simulink model "H2DFRL_LExCI_env_PPO"  (R2023a)
settings: Solver=FixedStepAuto  StartTime=0.0  StopTime=50  FixedStep=0.08  RelTol=1e-3
values from neighbouring files (symbols this model uses):
  action_mean_selector_ppo = 1:num_actions    [ReinforcementLearningBlockInit_H2DFRL.m]
  action_sampling_mode = 1    [ReinforcementLearningBlockInit_H2DFRL.m]
  action_selector_ddpg = 1:num_actions    [ReinforcementLearningBlockInit_H2DFRL.m]
  action_std_selector_ppo = 1:num_actions    [ReinforcementLearningBlockInit_H2DFRL.m]
  action_type = 1    [ReinforcementLearningBlockInit_H2DFRL.m]
  C2C_NMPC = init_C2C_NMPC_H2DF(C2C_NMPC.expdata)    [init_H2DFRL_GRU.m]
  LowerLimit = ([0.17e-3;350;-5;1e-3] - C2C_NMPC.Normalization.controls.mean)./(C2C_NMPC.Normalization.controls.std)    [init_H2DFRL_GRU.m]
  num_actions = 4    [ReinforcementLearningBlockInit_H2DFRL.m]
  rl_algorithm = 1    [ReinforcementLearningBlockInit_H2DFRL.m]
  UpperLimit = ([0.5e-3;900;2;5.5e-3] - C2C_NMPC.Normalization.controls.mean)./(C2C_NMPC.Normalization.controls.std)    [init_H2DFRL_GRU.m]
undefined symbols (not defined in the file or in its folder): CA50_offset, DiscIntNeverNeededParam, enable_CA50_noise, enable_CA50_offset, enable_IMEP_noise, enable_IMEP_offset, IMEP_offset, NUMBER_OF_ACTIONS
libraries: simulink x23, dspsrcs4 x4
(part 3 of 4)

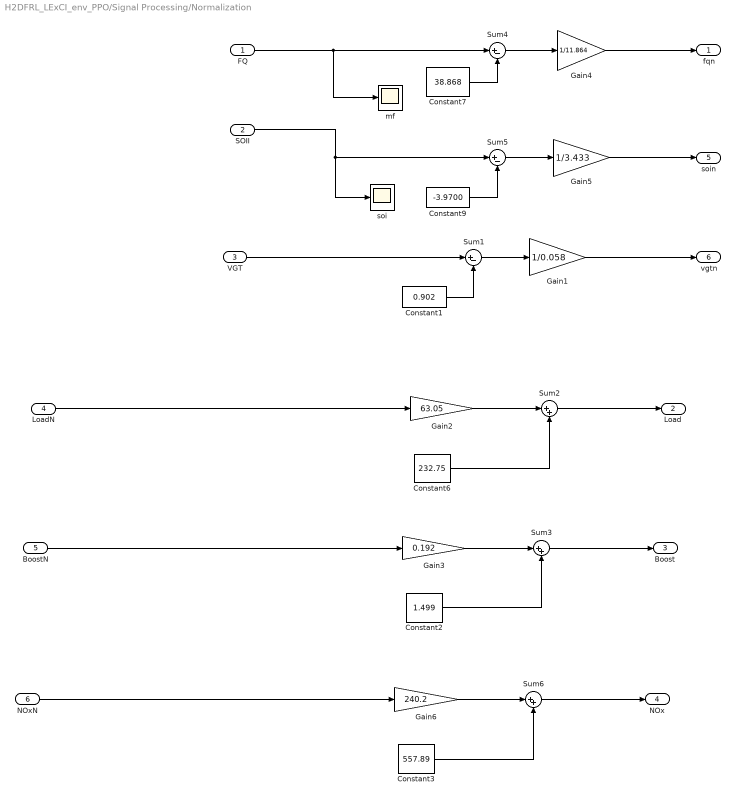
== system H2DFRL_LExCI_env_PPO/Signal Processing/Normalization ==
  FQ : Inport
  SOII : Inport  Port=2
  VGT : Inport  Port=3
  LoadN : Inport  Port=4
  BoostN : Inport  Port=5
  NOxN : Inport  Port=6
  Constant1 : Constant  Value=0.902
  Constant2 : Constant  Value=1.499
  Constant3 : Constant  Value=557.89
  Constant6 : Constant  Value=232.75
  Constant7 : Constant  Value=38.868
  Constant9 : Constant  Value=-3.9700
  Gain1 : Gain  Gain=1/0.058
  Gain2 : Gain  Gain=63.05
  Gain3 : Gain  Gain=0.192
  Gain4 : Gain  Gain=1/11.864
  Gain5 : Gain  Gain=1/3.433
  Gain6 : Gain  Gain=240.2
  Sum1 : Sum  Inputs=|+-
  Sum2 : Sum  Inputs=|++
  Sum3 : Sum  Inputs=|++
  Sum4 : Sum  Inputs=|+-
  Sum5 : Sum  Inputs=|+-
  Sum6 : Sum  Inputs=|++
  mf : Scope
  soi : Scope
  fqn : Outport
  Load : Outport  Port=2
  Boost : Outport  Port=3
  NOx : Outport  Port=4
  soin : Outport  Port=5
  vgtn : Outport  Port=6
  wires:
  Gain4/1 -> fqn/1
  SOII/1 -> soi/1, Sum5/1
  FQ/1 -> mf/1, Sum4/1
  Sum4/1 -> Gain4/1
  Gain5/1 -> soin/1
  Constant9/1 -> Sum5/2
  Sum5/1 -> Gain5/1
  Constant7/1 -> Sum4/2
  Sum1/1 -> Gain1/1
  Constant1/1 -> Sum1/2
  VGT/1 -> Sum1/1
  Gain1/1 -> vgtn/1
  Gain6/1 -> Sum6/1
  Sum6/1 -> NOx/1
  Sum2/1 -> Load/1
  NOxN/1 -> Gain6/1
  Constant3/1 -> Sum6/2
  Constant2/1 -> Sum3/2
  Gain3/1 -> Sum3/1
  Sum3/1 -> Boost/1
  Constant6/1 -> Sum2/2
  LoadN/1 -> Gain2/1
  BoostN/1 -> Gain3/1
  Gain2/1 -> Sum2/1

== system H2DFRL_LExCI_env_PPO/Signal Processing/calculate reward ==
  Reference : Inport
  controls : Inport  Port=2
  outputs : Inport  Port=3
  Gain : Gain  Gain=0.001
  Subsystem : Subsystem
  Unary Minus : UnaryMinus
  Unit Delay2 : UnitDelay  SampleTime=-1  HasFrameUpgradeWarning=on
  reward : Outport  VectorParamsAs1DForOutWhenUnconnected=off
  wires:
  Subsystem/1(Cost) -> Unary Minus/1
  Reference/1 -> Unit Delay2/1
  Unary Minus/1 -> Gain/1
  Gain/1 -> reward/1
  controls/1 -> Subsystem/2(controls)
  outputs/1 -> Subsystem/3(Outputs)
  Unit Delay2/1 -> Subsystem/1(Refernce)

== system H2DFRL_LExCI_env_PPO/Signal Processing/calculate reward1 ==
  Reference : Inport
  controls : Inport  Port=2
  outputs : Inport  Port=3
  Gain : Gain  Gain=0.001
  Subsystem : Subsystem
  Unary Minus : UnaryMinus
  Unit Delay2 : UnitDelay  SampleTime=-1  HasFrameUpgradeWarning=on
  reward : Outport  VectorParamsAs1DForOutWhenUnconnected=off
  wires:
  Subsystem/1(Cost) -> Unary Minus/1
  Reference/1 -> Unit Delay2/1
  Unary Minus/1 -> Gain/1
  Gain/1 -> reward/1
  controls/1 -> Subsystem/2(controls)
  outputs/1 -> Subsystem/3(Outputs)
  Unit Delay2/1 -> Subsystem/1(Refernce)

== system H2DFRL_LExCI_env_PPO/Signal Processing/generate observations1 ==
  Outputs : Inport
  Reference : Inport  Port=2
  LSTM States : Inport  Port=3
  Abs : Abs  SaturateOnIntegerOverflow=off
  Demux : Demux
  Demux1 : Demux
  Discrete-Time Integrator : DiscreteIntegrator  SampleTime=-1  ICPrevOutput=DiscIntNeverNeededParam  ICPrevScaledInput=DiscIntNeverNeededParam
  Display : Display
  Display1 : Display
  Display2 : Display
  Mux : Mux  Inputs=9
  Selector1 : Selector  IndexOptions=Index vector (dialog)  Indices=[1:4]  OutputSizes=1
  Subtract3 : Sum  Inputs=+-
  Unit Delay : UnitDelay  SampleTime=-1  HasFrameUpgradeWarning=on
  Unit Delay1 : UnitDelay  SampleTime=-1  HasFrameUpgradeWarning=on
  observations : Outport  VectorParamsAs1DForOutWhenUnconnected=off
  wires:
  Mux/1 -> observations/1, Display/1
  Demux1/1 -> Subtract3/2, Mux/1
  Demux1/2 -> Mux/2
  Demux1/3 -> Mux/3
  Demux1/4 -> Mux/4
  Subtract3/1 -> Mux/8, Discrete-Time Integrator/1
  Selector1/1 -> Demux/1, Display1/1
  Demux/1 -> Unit Delay/1, Unit Delay1/1, Mux/6
  Reference/1 -> Selector1/1
  LSTM States/1 -> Mux/9
  Outputs/1 -> Display2/1, Demux1/1
  Discrete-Time Integrator/1 -> Abs/1
  Unit Delay1/1 -> Subtract3/1
  Unit Delay/1 -> Mux/5
  Abs/1 -> Mux/7

== system H2DFRL_LExCI_env_PPO/Signal Processing/generate observations2 ==
  Outputs : Inport
  Reference : Inport  Port=2
  LSTM States : Inport  Port=3
  Demux : Demux
  Demux1 : Demux
  Display : Display
  Display1 : Display
  Display2 : Display
  Mux : Mux  Inputs=9
  Selector1 : Selector  IndexOptions=Index vector (dialog)  Indices=[1:4]  OutputSizes=1
  Subtract1 : Sum  Inputs=+-
  Subtract2 : Sum  Inputs=+-
  Subtract3 : Sum  Inputs=+-
  Unit Delay{,1..3} (4 alike) : UnitDelay  SampleTime=-1  HasFrameUpgradeWarning=on
  observations : Outport  VectorParamsAs1DForOutWhenUnconnected=off
  wires:
  Mux/1 -> observations/1, Display/1
  Demux1/1 -> Unit Delay3/1, Subtract2/1, Subtract3/2, Mux/1
  Demux1/4 -> Mux/4
  Subtract3/1 -> Mux/8
  Selector1/1 -> Demux/1, Display1/1
  Demux/1 -> Unit Delay/1, Unit Delay1/1, Mux/6
  Reference/1 -> Selector1/1
  LSTM States/1 -> Mux/9
  Outputs/1 -> Display2/1, Demux1/1
  Unit Delay1/1 -> Subtract3/1
  Unit Delay/1 -> Mux/5
  Demux1/2 -> Unit Delay2/1, Subtract1/1, Mux/2
  Unit Delay2/1 -> Subtract1/2
  Subtract1/1 -> Mux/3
  Unit Delay3/1 -> Subtract2/2
  Subtract2/1 -> Mux/7

== system H2DFRL_LExCI_env_PPO/Signal Processing/stop simulation ==
  Output : Inport
  Compare To Constant2 : simulink/Logic and Bit Operations/Compare To Constant  relop=<=  const=-100  OutDataTypeStr=boolean
  Demux : Demux
  stop : Outport  VectorParamsAs1DForOutWhenUnconnected=off
  wires:
  Demux/1 -> Compare To Constant2/1
  Compare To Constant2/1 -> stop/1
  Output/1 -> Demux/1

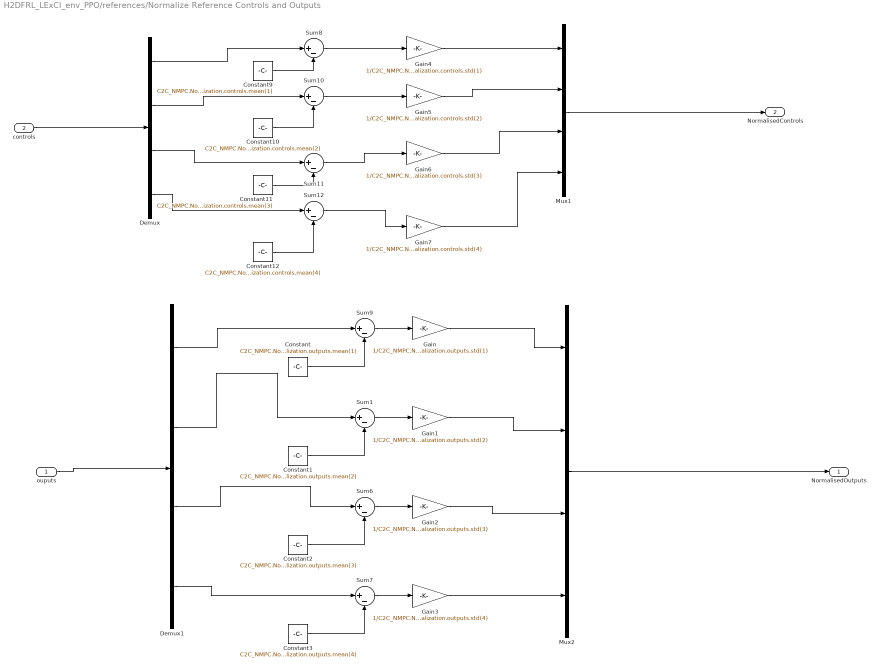
== system H2DFRL_LExCI_env_PPO/references/Normalize Reference Controls and Outputs ==
  "ouputs " : Inport
  controls : Inport  Port=2
  Constant : Constant  Value=C2C_NMPC.Normalization.outputs.mean(1)
  Constant1 : Constant  Value=C2C_NMPC.Normalization.outputs.mean(2)
  Constant10 : Constant  Value=C2C_NMPC.Normalization.controls.mean(2)
  Constant11 : Constant  Value=C2C_NMPC.Normalization.controls.mean(3)
  Constant12 : Constant  Value=C2C_NMPC.Normalization.controls.mean(4)
  Constant2 : Constant  Value=C2C_NMPC.Normalization.outputs.mean(3)
  Constant3 : Constant  Value=C2C_NMPC.Normalization.outputs.mean(4)
  Constant9 : Constant  Value=C2C_NMPC.Normalization.controls.mean(1)
  Demux : Demux
  Demux1 : Demux
  Gain : Gain  Gain=1/C2C_NMPC.Normalization.outputs.std(1)
  Gain1 : Gain  Gain=1/C2C_NMPC.Normalization.outputs.std(2)
  Gain2 : Gain  Gain=1/C2C_NMPC.Normalization.outputs.std(3)
  Gain3 : Gain  Gain=1/C2C_NMPC.Normalization.outputs.std(4)
  Gain4 : Gain  Gain=1/C2C_NMPC.Normalization.controls.std(1)
  Gain5 : Gain  Gain=1/C2C_NMPC.Normalization.controls.std(2)
  Gain6 : Gain  Gain=1/C2C_NMPC.Normalization.controls.std(3)
  Gain7 : Gain  Gain=1/C2C_NMPC.Normalization.controls.std(4)
  Mux1 : Mux
  Mux2 : Mux
  Sum{1,6..12} (8 alike) : Sum  Inputs=|+-
  NormalisedOutputs : Outport
  "NormalisedControls " : Outport  Port=2
  wires:
  Constant2/1 -> Sum6/2
  Gain7/1 -> Mux1/4
  Gain5/1 -> Mux1/2
  Constant12/1 -> Sum12/2
  Constant11/1 -> Sum11/2
  Gain4/1 -> Mux1/1
  Demux/1 -> Sum8/1
  Demux1/2 -> Sum1/1
  Constant/1 -> Sum9/2
  Sum11/1 -> Gain6/1
  Demux/4 -> Sum12/1
  Gain6/1 -> Mux1/3
  Constant1/1 -> Sum1/2
  Demux1/4 -> Sum7/1
  Demux1/3 -> Sum6/1
  Sum6/1 -> Gain2/1
  Sum9/1 -> Gain/1
  Sum10/1 -> Gain5/1
  Mux1/1 -> "NormalisedControls "/1
  Sum8/1 -> Gain4/1
  Sum12/1 -> Gain7/1
  Constant9/1 -> Sum8/2
  Demux/2 -> Sum10/1
  Constant10/1 -> Sum10/2
  Constant3/1 -> Sum7/2
  Sum1/1 -> Gain1/1
  Demux/3 -> Sum11/1
  Sum7/1 -> Gain3/1
  controls/1 -> Demux/1
  "ouputs "/1 -> Demux1/1
  Demux1/1 -> Sum9/1
  Gain1/1 -> Mux2/2
  Gain/1 -> Mux2/1
  Gain2/1 -> Mux2/3
  Gain3/1 -> Mux2/4
  Mux2/1 -> NormalisedOutputs/1

== system H2DFRL_LExCI_env_PPO/references/Subsystem1 ==
  Data Store Write : DataStoreWrite  DataStoreName=C2C_NMPC_IMEP_Weight  IndexOptions=Index vector (dialog)  Indices=1  OutputSizes=1
  Data Store Write1 : DataStoreWrite  DataStoreName=C2C_NMPC_NOX_Weight  IndexOptions=Index vector (dialog)  Indices=1  OutputSizes=1
  Data Store Write10 : DataStoreWrite  DataStoreName=C2C_NMPC_Delta_SOI_Main_Weight  IndexOptions=Index vector (dialog)  Indices=1  OutputSizes=1
  Data Store Write11 : DataStoreWrite  DataStoreName=C2C_NMPC_Delta_DOI_H2_Weight  IndexOptions=Index vector (dialog)  Indices=1  OutputSizes=1
  Data Store Write2 : DataStoreWrite  DataStoreName=C2C_NMPC_SOOT_Weight  IndexOptions=Index vector (dialog)  Indices=1  OutputSizes=1
  Data Store Write3 : DataStoreWrite  DataStoreName=C2C_NMPC_MPRR_Weight  IndexOptions=Index vector (dialog)  Indices=1  OutputSizes=1
  Data Store Write4 : DataStoreWrite  DataStoreName=C2C_NMPC_DOI_Main_Weight  IndexOptions=Index vector (dialog)  Indices=1  OutputSizes=1
  Data Store Write5 : DataStoreWrite  DataStoreName=C2C_NMPC_P2M_Weight  IndexOptions=Index vector (dialog)  Indices=1  OutputSizes=1
  Data Store Write6 : DataStoreWrite  DataStoreName=C2C_NMPC_SOI_Main_Weight  IndexOptions=Index vector (dialog)  Indices=1  OutputSizes=1
  Data Store Write7 : DataStoreWrite  DataStoreName=C2C_NMPC_DOI_H2_Weight  IndexOptions=Index vector (dialog)  Indices=1  OutputSizes=1
  Data Store Write8 : DataStoreWrite  DataStoreName=C2C_NMPC_Delta_DOI_Main_Weight  IndexOptions=Index vector (dialog)  Indices=1  OutputSizes=1
  Data Store Write9 : DataStoreWrite  DataStoreName=C2C_NMPC_Delta_P2M_Weight  IndexOptions=Index vector (dialog)  Indices=1  OutputSizes=1
  weight_IMEP : Constant  Value=10
  weight_Nox1 : Constant  Value=0
  weight_dt_u_{1..4} (4 alike) : Constant
  weight_mprr1 : Constant  Value=0
  weight_soot : Constant  Value=0
  weight_u_1 : Constant
  weight_u_2 : Constant  Value=0
  weight_u_3 : Constant  Value=0
  weight_u_4 : Constant
  wires:
  weight_soot/1 -> Data Store Write2/1
  weight_dt_u_4/1 -> Data Store Write11/1
  weight_dt_u_1/1 -> Data Store Write8/1
  weight_mprr1/1 -> Data Store Write3/1
  weight_dt_u_3/1 -> Data Store Write10/1
  weight_dt_u_2/1 -> Data Store Write9/1
  weight_Nox1/1 -> Data Store Write1/1
  weight_u_3/1 -> Data Store Write6/1
  weight_u_4/1 -> Data Store Write7/1
  weight_u_1/1 -> Data Store Write4/1
  weight_IMEP/1 -> Data Store Write/1
  weight_u_2/1 -> Data Store Write5/1

== system H2DFRL_LExCI_env_PPO/references/Subsystem4 ==
  C2C_NMPC_constraints_low_IMEP1 : Constant  Value=2.5e5
  C2C_NMPC_constraints_low_MPRR1 : Constant  Value=0
  C2C_NMPC_constraints_low_NOX1 : Constant  Value=0
  C2C_NMPC_constraints_low_SOOT1 : Constant  Value=0
  C2C_NMPC_constraints_up_IMEP1 : Constant  Value=12e5
  C2C_NMPC_constraints_up_MPRR1 : Constant  Value=5e5
  C2C_NMPC_constraints_up_NOX1 : Constant  Value=1000
  C2C_NMPC_constraints_up_SOOT1 : Constant  Value=5
  Data Store Write10 : DataStoreWrite  DataStoreName=C2C_NMPC_constraints_low_SOOT  IndexOptions=Index vector (dialog)  Indices=1  OutputSizes=1
  Data Store Write11 : DataStoreWrite  DataStoreName=C2C_NMPC_constraints_low_MPRR  IndexOptions=Index vector (dialog)  Indices=1  OutputSizes=1
  Data Store Write12 : DataStoreWrite  DataStoreName=C2C_NMPC_constraints_up_IMEP  IndexOptions=Index vector (dialog)  Indices=1  OutputSizes=1
  Data Store Write13 : DataStoreWrite  DataStoreName=C2C_NMPC_constraints_up_NOX  IndexOptions=Index vector (dialog)  Indices=1  OutputSizes=1
  Data Store Write14 : DataStoreWrite  DataStoreName=C2C_NMPC_constraints_up_SOOT  IndexOptions=Index vector (dialog)  Indices=1  OutputSizes=1
  Data Store Write15 : DataStoreWrite  DataStoreName=C2C_NMPC_constraints_up_MPRR  IndexOptions=Index vector (dialog)  Indices=1  OutputSizes=1
  Data Store Write8 : DataStoreWrite  DataStoreName=C2C_NMPC_constraints_low_IMEP  IndexOptions=Index vector (dialog)  Indices=1  OutputSizes=1
  Data Store Write9 : DataStoreWrite  DataStoreName=C2C_NMPC_constraints_low_NOX  IndexOptions=Index vector (dialog)  Indices=1  OutputSizes=1
  wires:
  C2C_NMPC_constraints_up_NOX1/1 -> Data Store Write13/1
  C2C_NMPC_constraints_up_IMEP1/1 -> Data Store Write12/1
  C2C_NMPC_constraints_up_SOOT1/1 -> Data Store Write14/1
  C2C_NMPC_constraints_up_MPRR1/1 -> Data Store Write15/1
  C2C_NMPC_constraints_low_MPRR1/1 -> Data Store Write11/1
  C2C_NMPC_constraints_low_NOX1/1 -> Data Store Write9/1
  C2C_NMPC_constraints_low_IMEP1/1 -> Data Store Write8/1
  C2C_NMPC_constraints_low_SOOT1/1 -> Data Store Write10/1

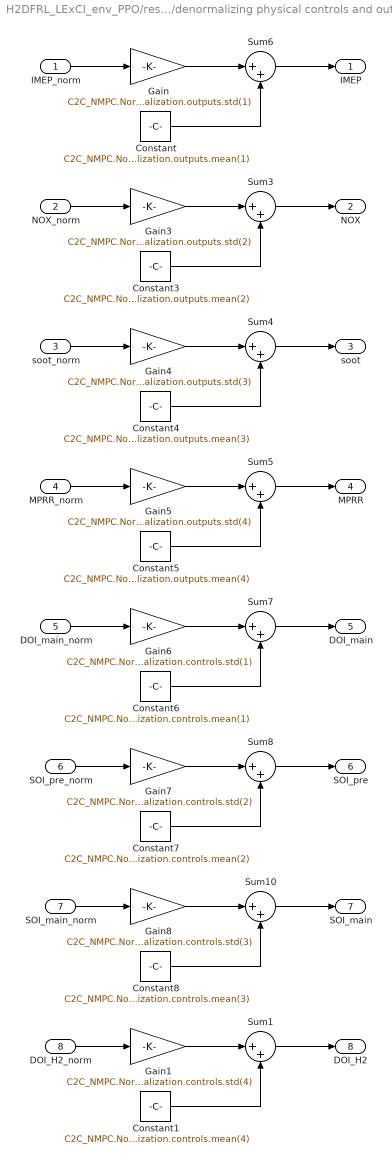
== system H2DFRL_LExCI_env_PPO/results/denormalizing physical controls and outputs ==
  IMEP_norm : Inport
  NOX_norm : Inport  Port=2
  soot_norm : Inport  Port=3
  MPRR_norm : Inport  Port=4
  DOI_main_norm : Inport  Port=5
  SOI_pre_norm : Inport  Port=6
  SOI_main_norm : Inport  Port=7
  DOI_H2_norm : Inport  Port=8
  Constant : Constant  Value=C2C_NMPC.Normalization.outputs.mean(1)
  Constant1 : Constant  Value=C2C_NMPC.Normalization.controls.mean(4)
  Constant3 : Constant  Value=C2C_NMPC.Normalization.outputs.mean(2)
  Constant4 : Constant  Value=C2C_NMPC.Normalization.outputs.mean(3)
  Constant5 : Constant  Value=C2C_NMPC.Normalization.outputs.mean(4)
  Constant6 : Constant  Value=C2C_NMPC.Normalization.controls.mean(1)
  Constant7 : Constant  Value=C2C_NMPC.Normalization.controls.mean(2)
  Constant8 : Constant  Value=C2C_NMPC.Normalization.controls.mean(3)
  Gain : Gain  Gain=C2C_NMPC.Normalization.outputs.std(1)
  Gain1 : Gain  Gain=C2C_NMPC.Normalization.controls.std(4)
  Gain3 : Gain  Gain=C2C_NMPC.Normalization.outputs.std(2)
  Gain4 : Gain  Gain=C2C_NMPC.Normalization.outputs.std(3)
  Gain5 : Gain  Gain=C2C_NMPC.Normalization.outputs.std(4)
  Gain6 : Gain  Gain=C2C_NMPC.Normalization.controls.std(1)
  Gain7 : Gain  Gain=C2C_NMPC.Normalization.controls.std(2)
  Gain8 : Gain  Gain=C2C_NMPC.Normalization.controls.std(3)
  Sum{1,3..8,10} (8 alike) : Sum  Inputs=|++
  IMEP : Outport
  NOX : Outport  Port=2
  soot : Outport  Port=3
  MPRR : Outport  Port=4
  DOI_main : Outport  Port=5
  SOI_pre : Outport  Port=6
  SOI_main : Outport  Port=7
  DOI_H2 : Outport  Port=8
  wires:
  Gain4/1 -> Sum4/1
  Constant3/1 -> Sum3/2
  Constant4/1 -> Sum4/2
  Gain3/1 -> Sum3/1
  Constant5/1 -> Sum5/2
  Gain5/1 -> Sum5/1
  Constant/1 -> Sum6/2
  Sum3/1 -> NOX/1
  NOX_norm/1 -> Gain3/1
  Sum5/1 -> MPRR/1
  Gain/1 -> Sum6/1
  IMEP_norm/1 -> Gain/1
  Sum6/1 -> IMEP/1
  MPRR_norm/1 -> Gain5/1
  Sum4/1 -> soot/1
  soot_norm/1 -> Gain4/1
  Constant7/1 -> Sum8/2
  Gain8/1 -> Sum10/1
  Constant6/1 -> Sum7/2
  Gain7/1 -> Sum8/1
  Sum10/1 -> SOI_main/1
  DOI_main_norm/1 -> Gain6/1
  Sum7/1 -> DOI_main/1
  Gain6/1 -> Sum7/1
  Sum8/1 -> SOI_pre/1
  Constant8/1 -> Sum10/2
  SOI_main_norm/1 -> Gain8/1
  SOI_pre_norm/1 -> Gain7/1
  DOI_H2_norm/1 -> Gain1/1
  Constant1/1 -> Sum1/2
  Gain1/1 -> Sum1/1
  Sum1/1 -> DOI_H2/1

== system H2DFRL_LExCI_env_PPO/results/denormalizing reference ==
  IMEP_norm : Inport
  NOX_norm : Inport  Port=2
  soot_norm : Inport  Port=3
  MPRR_norm : Inport  Port=4
  Constant : Constant  Value=C2C_NMPC.Normalization.outputs.mean(1)
  Constant1 : Constant  Value=C2C_NMPC.Normalization.outputs.mean(2)
  Constant2 : Constant  Value=C2C_NMPC.Normalization.outputs.mean(3)
  Constant3 : Constant  Value=C2C_NMPC.Normalization.outputs.mean(4)
  Gain : Gain  Gain=C2C_NMPC.Normalization.outputs.std(1)
  Gain1 : Gain  Gain=C2C_NMPC.Normalization.outputs.std(2)
  Gain2 : Gain  Gain=C2C_NMPC.Normalization.outputs.std(3)
  Gain3 : Gain  Gain=C2C_NMPC.Normalization.outputs.std(4)
  Sum{1..3,5} (4 alike) : Sum  Inputs=|++
  IMEP : Outport
  NOX : Outport  Port=2
  soot : Outport  Port=3
  MPRR : Outport  Port=4
  wires:
  Gain/1 -> Sum5/1
  IMEP_norm/1 -> Gain/1
  Constant/1 -> Sum5/2
  Sum5/1 -> IMEP/1
  Gain1/1 -> Sum1/1
  Constant1/1 -> Sum1/2
  NOX_norm/1 -> Gain1/1
  Sum1/1 -> NOX/1
  Gain2/1 -> Sum2/1
  Constant2/1 -> Sum2/2
  soot_norm/1 -> Gain2/1
  Sum2/1 -> soot/1
  Gain3/1 -> Sum3/1
  Constant3/1 -> Sum3/2
  MPRR_norm/1 -> Gain3/1
  Sum3/1 -> MPRR/1

== system H2DFRL_LExCI_env_PPO/Engine Model/offset_and_noise/CA50_generation ==
  CA50_in : Inport
  Add : Sum
  Add1 : Sum
  Band-Limited White Noise : simulink/Sources/Band-Limited White Noise  Cov=0.01  Ts=1  seed=[23341]
  Constant1 : Constant  Value=CA50_offset
  Constant2 : Constant  Value=0
  Constant3 : Constant  Value=enable_CA50_noise
  Constant4 : Constant  Value=0
  Constant5 : Constant  Value=enable_CA50_offset
  Switch1 : Switch  Criteria=u2 > Threshold  SaturateOnIntegerOverflow=off  InputSameDT=off
  Switch2 : Switch  Criteria=u2 > Threshold  SaturateOnIntegerOverflow=off  InputSameDT=off
  denormalizing_CA50 : Subsystem
  normalizing_CA50 : Subsystem
  CA50_out : Outport
  wires:
  Add/1 -> Add1/2
  Switch1/1 -> Add1/1
  Constant4/1 -> Switch1/3
  Constant3/1 -> Switch1/2
  Band-Limited White Noise/1 -> Switch1/1
  CA50_in/1 -> denormalizing_CA50/1(CA50_in)
  denormalizing_CA50/1(CA50) -> Add/2
  Switch2/1 -> Add/1
  Constant1/1 -> Switch2/1
  Constant5/1 -> Switch2/2
  Constant2/1 -> Switch2/3
  normalizing_CA50/1(CA50_out) -> CA50_out/1
  Add1/1 -> normalizing_CA50/1(CA50)

== system H2DFRL_LExCI_env_PPO/Engine Model/offset_and_noise/IMEP_generation ==
  IMEP_in : Inport
  Add : Sum
  Add1 : Sum
  Band-Limited White Noise : simulink/Sources/Band-Limited White Noise  Cov=0.01  Ts=1  seed=[23341]
  Constant1 : Constant  Value=IMEP_offset
  Constant2 : Constant  Value=0
  Constant3 : Constant  Value=enable_IMEP_noise
  Constant4 : Constant  Value=0
  Constant5 : Constant  Value=enable_IMEP_offset
  Switch1 : Switch  Criteria=u2 > Threshold  SaturateOnIntegerOverflow=off  InputSameDT=off
  Switch2 : Switch  Criteria=u2 > Threshold  SaturateOnIntegerOverflow=off  InputSameDT=off
  denormalizing_IMEP : Subsystem
  normalizing_IMEP : Subsystem
  IMEP_out : Outport
  wires:
  Add/1 -> Add1/2
  Switch1/1 -> Add1/1
  Constant4/1 -> Switch1/3
  Constant3/1 -> Switch1/2
  Band-Limited White Noise/1 -> Switch1/1
  IMEP_in/1 -> denormalizing_IMEP/1(IMEP_in)
  denormalizing_IMEP/1(IMEP) -> Add/2
  Switch2/1 -> Add/1
  Constant1/1 -> Switch2/1
  Constant5/1 -> Switch2/2
  Constant2/1 -> Switch2/3
  normalizing_IMEP/1(IMEP_out) -> IMEP_out/1
  Add1/1 -> normalizing_IMEP/1(IMEP)

== system H2DFRL_LExCI_env_PPO/Engine Model/offset_and_noise1/IMEP_generation ==
  IMEP_in : Inport
  Add : Sum
  Add1 : Sum
  Add2 : Sum  Inputs=+-
  Band-Limited White Noise : simulink/Sources/Band-Limited White Noise  Cov=0.1  Ts=0.08  seed=[23341]
  Constant1 : Constant  Commented=on  Value=IMEP_offset
  Constant2 : Constant  Value=0
  Constant3 : Constant
  Constant4 : Constant  Value=0
  Constant5 : Constant
  Constant6 : Constant  Value=0
  Display : Display
  Gain : Gain  Gain=10000
  Scope : Scope  NumInputPorts=2
  Scope1 : Scope
  Switch1 : Switch  Criteria=u2 > Threshold  SaturateOnIntegerOverflow=off  InputSameDT=off
  Switch2 : Switch  Criteria=u2 > Threshold  SaturateOnIntegerOverflow=off  InputSameDT=off
  denormalizing_IMEP : Subsystem
  normalizing_IMEP : Subsystem
  IMEP_out : Outport
  wires:
  Add/1 -> Add1/2
  Switch1/1 -> Display/1, Add1/1
  Constant4/1 -> Switch1/3
  Constant3/1 -> Switch1/2
  Band-Limited White Noise/1 -> Gain/1
  denormalizing_IMEP/1(IMEP) -> Add/2
  Switch2/1 -> Add/1
  Constant5/1 -> Switch2/2
  Constant2/1 -> Switch2/3
  normalizing_IMEP/1(IMEP_out) -> IMEP_out/1
  Add1/1 -> Add2/1, Scope/2, normalizing_IMEP/1(IMEP)
  Constant6/1 -> Switch2/1
  Gain/1 -> Switch1/1
  IMEP_in/1 -> Scope/1, Add2/2, denormalizing_IMEP/1(IMEP_in)
  Add2/1 -> Scope1/1

== system H2DFRL_LExCI_env_PPO/RL_Block/RL_Agent/Denormalization ==
  norm_action : Inport
  lower_action_bounds : Inport  Port=2
  upper_action_bounds : Inport  Port=3
  action_sampling_mode_selector : Inport  Port=4
  Add : Sum
  Constant : Constant  OutDataTypeStr=single
  Constant1 : Constant  Value=2  OutDataTypeStr=single
  Data Type Conversion : DataTypeConversion  SaturateOnIntegerOverflow=off  RndMeth=Floor
  Data Type Conversion1 : DataTypeConversion  SaturateOnIntegerOverflow=off  RndMeth=Floor
  Divide : Product  Inputs=*/
  Ground : Ground
  Multiport Switch : MultiPortSwitch  SaturateOnIntegerOverflow=off  InputSameDT=off
  Product : Product
  Saturation : Saturate  UpperLimit=1  LowerLimit=-1
  Subtract : Sum  Inputs=+-
  Subtract1 : Sum
  Tanh : Trigonometry  Operator=tanh
  action : Outport
  wires:
  action_sampling_mode_selector/1 -> Multiport Switch/1
  upper_action_bounds/1 -> Subtract/1
  Multiport Switch/1 -> Add/1
  lower_action_bounds/1 -> Subtract/2, Subtract1/2
  Add/1 -> Divide/1
  Subtract1/1 -> Data Type Conversion/1
  Divide/1 -> Product/1
  Product/1 -> Data Type Conversion1/1
  Constant1/1 -> Divide/2
  Constant/1 -> Add/2
  Tanh/1 -> Multiport Switch/2
  Subtract/1 -> Product/2
  norm_action/1 -> Saturation/1, Tanh/1
  Saturation/1 -> Multiport Switch/3
  Ground/1 -> Multiport Switch/4
  Data Type Conversion/1 -> action/1
  Data Type Conversion1/1 -> Subtract1/1

== system H2DFRL_LExCI_env_PPO/RL_Block/RL_Agent/Experience Buffer ==
  norm_observation : Inport
  norm_action : Inport  Port=2
  reward : Inport  Port=3
  new_norm_observation : Inport  Port=4
  b_episode_finished : Inport  Port=5
  Bus Creator : BusCreator  Inputs=5
  Data Type Conversion3 : DataTypeConversion  OutDataTypeStr=single  SaturateOnIntegerOverflow=off  RndMeth=Floor
  Terminator : Terminator
  To Workspace : ToWorkspace  VariableName=norm_obs  SampleTime=-1
  To Workspace1 : ToWorkspace  VariableName=norm_action  SampleTime=-1
  To Workspace2 : ToWorkspace  VariableName=reward  SampleTime=-1
  To Workspace3 : ToWorkspace  VariableName=new_norm_obs  SampleTime=-1
  To Workspace4 : ToWorkspace  VariableName=done  SampleTime=-1
  Unit Delay : UnitDelay  SampleTime=-1  HasFrameUpgradeWarning=on
  b_episode_finished_out : Gain  OutDataTypeStr=Inherit: Same as input
  b_episode_finished_terminate_episode : Gain  OutDataTypeStr=Inherit: Same as input
  new_norm_observation_out : Gain  OutDataTypeStr=Inherit: Same as input
  norm_action_out : Gain  OutDataTypeStr=Inherit: Same as input
  norm_observation_out : Gain  OutDataTypeStr=Inherit: Same as input
  reward_out : Gain  OutDataTypeStr=Inherit: Same as input
  Experience Tuple : Outport
  wires:
  b_episode_finished_terminate_episode/1 -> Terminator/1
  Unit Delay/1 -> b_episode_finished_terminate_episode/1
  b_episode_finished_out/1 -> To Workspace4/1, Bus Creator/5
  reward_out/1 -> To Workspace2/1, Bus Creator/3
  norm_action_out/1 -> To Workspace1/1, Bus Creator/2
  norm_observation_out/1 -> To Workspace/1, Bus Creator/1
  Data Type Conversion3/1 -> b_episode_finished_out/1
  Bus Creator/1 -> Experience Tuple/1
  b_episode_finished/1 -> Data Type Conversion3/1, Unit Delay/1
  reward/1 -> reward_out/1
  norm_action/1 -> norm_action_out/1
  norm_observation/1 -> norm_observation_out/1
  new_norm_observation/1 -> new_norm_observation_out/1
  new_norm_observation_out/1 -> To Workspace3/1, Bus Creator/4

== system H2DFRL_LExCI_env_PPO/RL_Block/RL_Agent/Normalization ==
  observation : Inport
  lower_observation_bounds : Inport  Port=2
  upper_observation_bounds : Inport  Port=3
  Constant : Constant
  Data Type Conversion : DataTypeConversion  OutDataTypeStr=single  SaturateOnIntegerOverflow=off  RndMeth=Floor
  Divide : Product  Inputs=*/
  Gain : Gain  Gain=2
  Saturation : Saturate  UpperLimit=1  LowerLimit=-1
  Subtract : Sum  Inputs=+-
  Subtract1 : Sum  Inputs=-+
  Subtract2 : Sum  Inputs=+-
  norm_observation : Outport
  wires:
  Saturation/1 -> Data Type Conversion/1
  lower_observation_bounds/1 -> Subtract1/1, Subtract/2
  upper_observation_bounds/1 -> Subtract1/2
  observation/1 -> Subtract/1
  Data Type Conversion/1 -> norm_observation/1
  Divide/1 -> Gain/1
  Subtract1/1 -> Divide/2
  Subtract/1 -> Divide/1
  Gain/1 -> Subtract2/1
  Subtract2/1 -> Saturation/1
  Constant/1 -> Subtract2/2

== system H2DFRL_LExCI_env_PPO/RL_Block/RL_Agent/Sampling ==
  norm_action_dist : Inport
  b_training_active : Inport  Port=2
  rl_algorithm : Inport  Port=3
  action_type_selector : Inport  Port=4
  ddpg_standard_deviation : Inport  Port=5
  Cast To Single : DataTypeConversion  OutDataTypeStr=single  SaturateOnIntegerOverflow=off  RndMeth=Floor
  Compare To Constant : simulink/Logic and Bit Operations/Compare To Constant  relop===  const=1  OutDataTypeStr=boolean
  Compare To Constant1 : simulink/Logic and Bit Operations/Compare To Constant  relop===  const=2  OutDataTypeStr=boolean
  Continuous Action : Subsystem
  Data Type Conversion : DataTypeConversion  OutDataTypeStr=single  SaturateOnIntegerOverflow=off  RndMeth=Floor
  Discrete Action : Subsystem
  Switch2 : Switch  Criteria=u2 > Threshold  Threshold=1.5  OutDataTypeStr=single  SaturateOnIntegerOverflow=off  InputSameDT=off
  norm_action : Outport
  wires:
  Continuous Action/1("norm_action ") -> Switch2/3
  Switch2/1 -> Data Type Conversion/1
  Compare To Constant/1 -> Continuous Action/Enable
  norm_action_dist/1 -> Continuous Action/1(norm_action_dist), Discrete Action/1(norm_action_dist)
  action_type_selector/1 -> Compare To Constant1/1, Compare To Constant/1, Cast To Single/1
  Compare To Constant1/1 -> Discrete Action/Enable
  Discrete Action/1("norm_action ") -> Switch2/1
  b_training_active/1 -> Continuous Action/2(b_training_active), Discrete Action/2(b_training_active)
  rl_algorithm/1 -> Discrete Action/3(rl_algorithm_selector), Continuous Action/3(rl_algorithm_selector)
  ddpg_standard_deviation/1 -> Continuous Action/4(ddpg_standard_deviation)
  Cast To Single/1 -> Switch2/2
  Data Type Conversion/1 -> norm_action/1

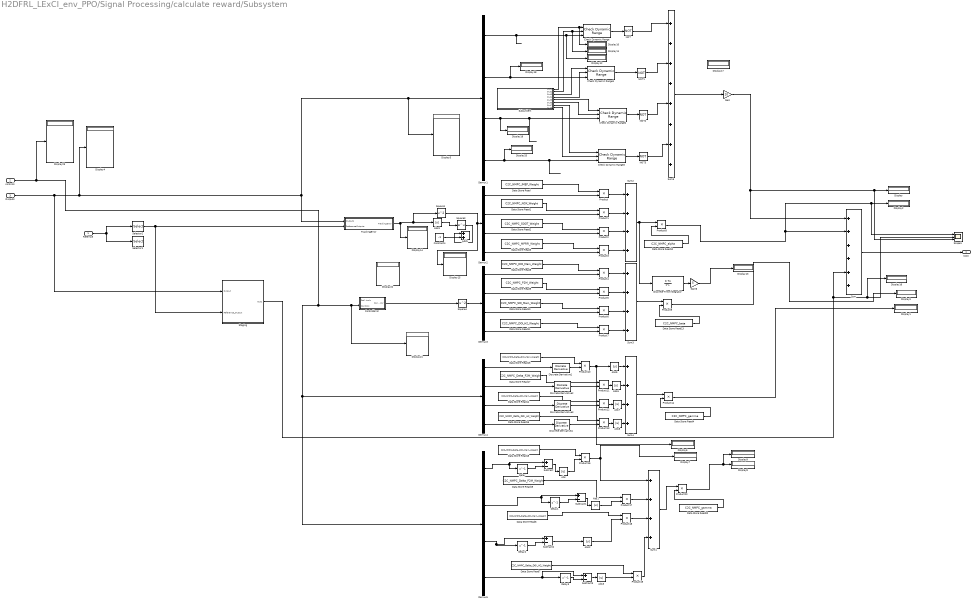
== system H2DFRL_LExCI_env_PPO/Signal Processing/calculate reward/Subsystem ==
  Refernce : Inport
  controls : Inport  Port=2
  Outputs : Inport  Port=3
  Abs{,1..3,5..9} (9 alike) : Abs  SaturateOnIntegerOverflow=off
  Add1 : Sum
  Check Dynamic Range{,1..3} (4 alike) : simulink/Model Verification/Check  Dynamic Range  Description=min < u < max  enabled=off  stopWhenAssertionFail=off  export=on  icon=graphic
  Constant4 : Constant  Value=-1
  ControlError : Subsystem
  Data Store Read : DataStoreRead  DataStoreName=C2C_NMPC_IMEP_Weight  IndexOptions=Index vector (dialog)  Indices=1  OutputSizes=1
  Data Store Read1 : DataStoreRead  DataStoreName=C2C_NMPC_NOX_Weight  IndexOptions=Index vector (dialog)  Indices=1  OutputSizes=1
  Data Store Read10 : DataStoreRead  DataStoreName=C2C_NMPC_SOI_Main_Weight  IndexOptions=Index vector (dialog)  Indices=1  OutputSizes=1
  Data Store Read11 : DataStoreRead  DataStoreName=C2C_NMPC_DOI_H2_Weight  IndexOptions=Index vector (dialog)  Indices=1  OutputSizes=1
  Data Store Read12 : DataStoreRead  DataStoreName=C2C_NMPC_alpha  IndexOptions=Index vector (dialog)  Indices=1  OutputSizes=1
  Data Store Read13 : DataStoreRead  DataStoreName=C2C_NMPC_beta  IndexOptions=Index vector (dialog)  Indices=1  OutputSizes=1
  Data Store Read14 : DataStoreRead  DataStoreName=C2C_NMPC_Delta_SOI_Main_Weight  IndexOptions=Index vector (dialog)  Indices=1  OutputSizes=1
  Data Store Read15 : DataStoreRead  DataStoreName=C2C_NMPC_Delta_DOI_H2_Weight  IndexOptions=Index vector (dialog)  Indices=1  OutputSizes=1
  Data Store Read16 : DataStoreRead  DataStoreName=C2C_NMPC_Delta_DOI_Main_Weight  IndexOptions=Index vector (dialog)  Indices=1  OutputSizes=1
  Data Store Read17 : DataStoreRead  DataStoreName=C2C_NMPC_Delta_P2M_Weight  IndexOptions=Index vector (dialog)  Indices=1  OutputSizes=1
  Data Store Read18 : DataStoreRead  DataStoreName=C2C_NMPC_Delta_DOI_Main_Weight  IndexOptions=Index vector (dialog)  Indices=1  OutputSizes=1
  Data Store Read19 : DataStoreRead  DataStoreName=C2C_NMPC_Delta_P2M_Weight  IndexOptions=Index vector (dialog)  Indices=1  OutputSizes=1
  Data Store Read2 : DataStoreRead  DataStoreName=C2C_NMPC_SOOT_Weight  IndexOptions=Index vector (dialog)  Indices=1  OutputSizes=1
  Data Store Read20 : DataStoreRead  DataStoreName=C2C_NMPC_gamma  IndexOptions=Index vector (dialog)  Indices=1  OutputSizes=1
  Data Store Read3 : DataStoreRead  DataStoreName=C2C_NMPC_MPRR_Weight  IndexOptions=Index vector (dialog)  Indices=1  OutputSizes=1
  Data Store Read4 : DataStoreRead  DataStoreName=C2C_NMPC_gamma  IndexOptions=Index vector (dialog)  Indices=1  OutputSizes=1
  Data Store Read6 : DataStoreRead  DataStoreName=C2C_NMPC_Delta_SOI_Main_Weight  IndexOptions=Index vector (dialog)  Indices=1  OutputSizes=1
  Data Store Read7 : DataStoreRead  DataStoreName=C2C_NMPC_Delta_DOI_H2_Weight  IndexOptions=Index vector (dialog)  Indices=1  OutputSizes=1
  Data Store Read8 : DataStoreRead  DataStoreName=C2C_NMPC_DOI_Main_Weight  IndexOptions=Index vector (dialog)  Indices=1  OutputSizes=1
  Data Store Read9 : DataStoreRead  DataStoreName=C2C_NMPC_P2M_Weight  IndexOptions=Index vector (dialog)  Indices=1  OutputSizes=1
  Delay{,1..3} (4 alike) : Delay  DelayLength=1
  Demux{1..5} (5 alike) : Demux
  Discrete Derivative{1..4} (4 alike) : simulink/Discrete/Discrete Derivative  gainval=1.0  ICPrevScaledInput=0.0  OutMin=[]  OutMax=[]  OutDataType=fixdt(1, 16)  OutScaling=2^-10  DoSatur=off
  Discrete-Time Integrator : DiscreteIntegrator  SampleTime=-1  ICPrevOutput=DiscIntNeverNeededParam  ICPrevScaledInput=DiscIntNeverNeededParam
  Display{,1..23} (24 alike) : Display
  Gain : Gain  Gain=20
  Gain6 : Gain  Gain=5
  NOT{,1..3} (4 alike) : Logic  Operator=NOT  IconShape=distinctive  AllPortsSameDT=off  OutDataTypeStr=boolean
  Product{,1..14,16..20} (20 alike) : Product
  Scope1 : Scope  NumInputPorts=3
  Selector1 : Selector  IndexOptions=Index vector (dialog)  Indices=[5:8]  OutputSizes=1
  Selector2 : Selector  IndexOptions=Index vector (dialog)  Indices=[1:4]  OutputSizes=1
  Square1 : Math  Operator=square  SignedPower=on
  Square3 : Math  SignedPower=on
  Square4 : Math  Operator=square  SignedPower=on
  Staging : Subsystem
  Subsystem : Subsystem
  Subtract{,1..3} (4 alike) : Sum  Inputs=+-
  Sum : Sum  Inputs=++++++
  Sum{1..4} (4 alike) : Sum  Inputs=++++
  Sum5 : Sum  Inputs=++++++++
  TrackingError : Subsystem
  Cost : Outport  VectorParamsAs1DForOutWhenUnconnected=off
  wires:
  Sum/1 -> Cost/1
  Outputs/1 -> Display5/1, Demux1/1, TrackingError/1(Outputs), Display4/1, Staging/1(Output)
  Data Store Read/1 -> Product/1
  Demux2/1 -> Product/2
  Demux2/2 -> Product1/2
  Data Store Read1/1 -> Product1/1
  Demux2/3 -> Product2/2
  Data Store Read2/1 -> Product2/1
  Demux2/4 -> Product3/2
  Data Store Read3/1 -> Product3/1
  Product2/1 -> Sum2/3
  Product1/1 -> Sum2/2
  Product/1 -> Sum2/1
  Product3/1 -> Sum2/4
  TrackingError/1(TrackingError) -> Square1/1, Abs9/1, Display14/1
  Product4/1 -> Sum3/1
  Data Store Read10/1 -> Product6/1
  Product7/1 -> Sum3/4
  Product5/1 -> Sum3/2
  Demux3/3 -> Product6/2
  Data Store Read8/1 -> Product4/1
  Demux3/4 -> Product7/2
  ControlError/1(ControlError) -> Square4/1
  Data Store Read9/1 -> Product5/1
  Product6/1 -> Sum3/3
  Demux3/1 -> Product4/2
  Demux3/2 -> Product5/2
  Data Store Read11/1 -> Product7/1
  Sum2/1 -> Discrete-Time Integrator/1, Product8/1
  Data Store Read12/1 -> Product8/2
  Sum3/1 -> Product9/1
  Data Store Read13/1 -> Product9/2
  Square4/1 -> Demux3/1
  Data Store Read17/1 -> Product11/1
  Data Store Read15/1 -> Product13/1
  Demux4/2 -> Discrete Derivative2/1
  Demux4/1 -> Discrete Derivative1/1
  Product12/1 -> Abs7/1
  Product10/1 -> Display6/1, Abs5/1
  Product13/1 -> Abs8/1
  Demux4/4 -> Discrete Derivative4/1
  Demux4/3 -> Discrete Derivative3/1
  Data Store Read16/1 -> Product10/1
  Data Store Read14/1 -> Product12/1
  Product11/1 -> Abs6/1
  Discrete Derivative1/1 -> Product10/2
  Discrete Derivative2/1 -> Product11/2
  Discrete Derivative3/1 -> Product12/2
  Discrete Derivative4/1 -> Product13/2
  Data Store Read4/1 -> Product14/2
  Sum4/1 -> Product14/1
  Demux1/1 -> Display12/1, Check Dynamic Range/3
  Check Dynamic Range/1 -> NOT/1
  Check Dynamic Range1/1 -> NOT1/1
  Check Dynamic Range2/1 -> NOT2/1
  Check Dynamic Range3/1 -> NOT3/1
  Sum5/1 -> Gain/1
  Product8/1 -> Scope1/1, Display2/1, Sum/2
  Product20/1 -> Display9/1, Display8/1
  Product9/1 -> Display3/1
  Refernce/1 -> Selector2/1, Selector1/1
  Selector2/1 -> Staging/2(Reference_Output), TrackingError/2(ReferenceOutputs)
  Subsystem/1(Out1) -> Display10/1, Check Dynamic Range/1
  Subsystem/2(Out2) -> Display11/1, Check Dynamic Range/2
  Subsystem/3(Out3) -> Check Dynamic Range1/1
  Subsystem/4(Out4) -> Check Dynamic Range1/2
  Subsystem/5(Out5) -> Check Dynamic Range2/1
  Subsystem/6(Out6) -> Check Dynamic Range2/2
  Subsystem/7(Out7) -> Check Dynamic Range3/1
  Subsystem/8(Out8) -> Check Dynamic Range3/2
  Product19/1 -> Sum1/4
  Product16/1 -> Display7/1, Sum1/1
  Abs/1 -> Product16/2
  Product18/1 -> Sum1/3
  Demux5/1 -> Subtract/1, Delay/1
  Product17/1 -> Sum1/2
  Data Store Read7/1 -> Product19/1
  Data Store Read6/1 -> Product18/1
  Abs3/1 -> Product19/2
  Data Store Read19/1 -> Product17/1
  Data Store Read18/1 -> Product16/1
  Sum1/1 -> Product20/1
  Data Store Read20/1 -> Product20/2
  Delay/1 -> Subtract/2
  Subtract/1 -> Abs/1
  Subtract1/1 -> Abs1/1
  Delay1/1 -> Subtract1/2
  Demux5/2 -> Subtract1/1, Delay1/1
  Abs1/1 -> Product17/2
  Demux5/3 -> Subtract2/1, Delay2/1
  Delay2/1 -> Subtract2/2
  Subtract2/1 -> Abs2/1
  Abs2/1 -> Product18/2
  Demux5/4 -> Subtract3/1, Delay3/1
  Delay3/1 -> Subtract3/2
  Subtract3/1 -> Abs3/1
  Product14/1 -> Display1/1
  controls/1 -> Display23/1, Demux4/1, Demux5/1, Display21/1, ControlError/2(Controls)
  NOT/1 -> Sum5/1
  NOT1/1 -> Sum5/3
  NOT2/1 -> Sum5/5
  NOT3/1 -> Sum5/7
  Abs5/1 -> Sum4/1
  Abs6/1 -> Sum4/2
  Abs7/1 -> Sum4/3
  Abs8/1 -> Sum4/4
  Gain/1 -> Sum/1, Scope1/3, Display/1
  Discrete-Time Integrator/1 -> Gain6/1
  Gain6/1 -> Display13/1
  Constant4/1 -> Add1/2
  Abs9/1 -> Square3/1
  Square3/1 -> Add1/1
  Square1/1 -> Display15/1, Demux2/1
  ? -> ?
  ? -> Display17/1, Sum5/2
  Demux1/2 -> Display18/1, Check Dynamic Range1/3
  Demux1/3 -> Check Dynamic Range2/3, Display19/1
  ? -> Sum5/6
  Demux1/4 -> Check Dynamic Range3/3, Display20/1
  Staging/1(Out1) -> Scope1/2, Display16/1, Sum/5

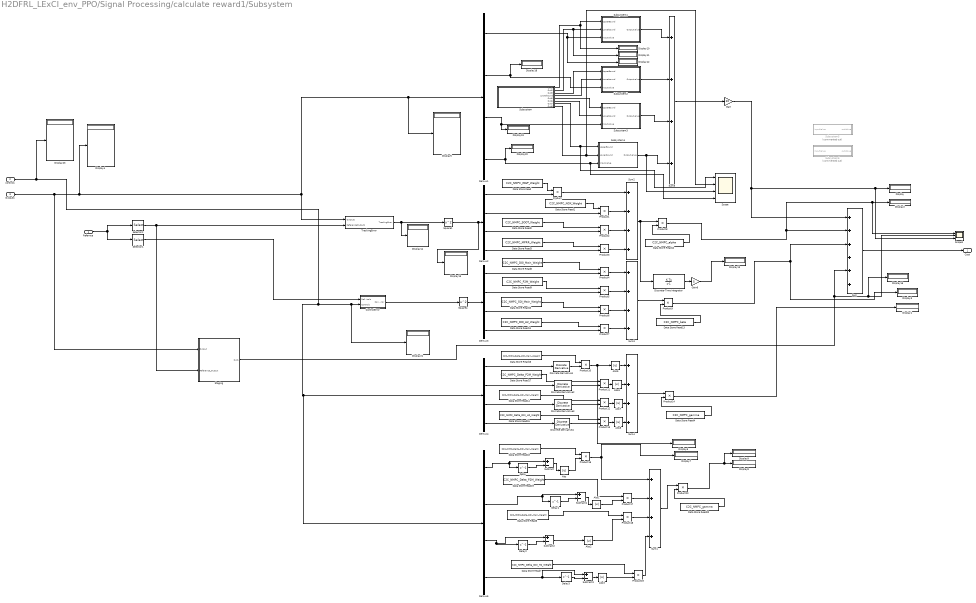
== system H2DFRL_LExCI_env_PPO/Signal Processing/calculate reward1/Subsystem ==
  Refernce : Inport
  controls : Inport  Port=2
  Outputs : Inport  Port=3
  Abs{,1..3,5..8} (8 alike) : Abs  SaturateOnIntegerOverflow=off
  ControlError : Subsystem
  Data Store Read : DataStoreRead  DataStoreName=C2C_NMPC_IMEP_Weight  IndexOptions=Index vector (dialog)  Indices=1  OutputSizes=1
  Data Store Read1 : DataStoreRead  DataStoreName=C2C_NMPC_NOX_Weight  IndexOptions=Index vector (dialog)  Indices=1  OutputSizes=1
  Data Store Read10 : DataStoreRead  DataStoreName=C2C_NMPC_SOI_Main_Weight  IndexOptions=Index vector (dialog)  Indices=1  OutputSizes=1
  Data Store Read11 : DataStoreRead  DataStoreName=C2C_NMPC_DOI_H2_Weight  IndexOptions=Index vector (dialog)  Indices=1  OutputSizes=1
  Data Store Read12 : DataStoreRead  DataStoreName=C2C_NMPC_alpha  IndexOptions=Index vector (dialog)  Indices=1  OutputSizes=1
  Data Store Read13 : DataStoreRead  DataStoreName=C2C_NMPC_beta  IndexOptions=Index vector (dialog)  Indices=1  OutputSizes=1
  Data Store Read14 : DataStoreRead  DataStoreName=C2C_NMPC_Delta_SOI_Main_Weight  IndexOptions=Index vector (dialog)  Indices=1  OutputSizes=1
  Data Store Read15 : DataStoreRead  DataStoreName=C2C_NMPC_Delta_DOI_H2_Weight  IndexOptions=Index vector (dialog)  Indices=1  OutputSizes=1
  Data Store Read16 : DataStoreRead  DataStoreName=C2C_NMPC_Delta_DOI_Main_Weight  IndexOptions=Index vector (dialog)  Indices=1  OutputSizes=1
  Data Store Read17 : DataStoreRead  DataStoreName=C2C_NMPC_Delta_P2M_Weight  IndexOptions=Index vector (dialog)  Indices=1  OutputSizes=1
  Data Store Read18 : DataStoreRead  DataStoreName=C2C_NMPC_Delta_DOI_Main_Weight  IndexOptions=Index vector (dialog)  Indices=1  OutputSizes=1
  Data Store Read19 : DataStoreRead  DataStoreName=C2C_NMPC_Delta_P2M_Weight  IndexOptions=Index vector (dialog)  Indices=1  OutputSizes=1
  Data Store Read2 : DataStoreRead  DataStoreName=C2C_NMPC_SOOT_Weight  IndexOptions=Index vector (dialog)  Indices=1  OutputSizes=1
  Data Store Read20 : DataStoreRead  DataStoreName=C2C_NMPC_gamma  IndexOptions=Index vector (dialog)  Indices=1  OutputSizes=1
  Data Store Read3 : DataStoreRead  DataStoreName=C2C_NMPC_MPRR_Weight  IndexOptions=Index vector (dialog)  Indices=1  OutputSizes=1
  Data Store Read4 : DataStoreRead  DataStoreName=C2C_NMPC_gamma  IndexOptions=Index vector (dialog)  Indices=1  OutputSizes=1
  Data Store Read6 : DataStoreRead  DataStoreName=C2C_NMPC_Delta_SOI_Main_Weight  IndexOptions=Index vector (dialog)  Indices=1  OutputSizes=1
  Data Store Read7 : DataStoreRead  DataStoreName=C2C_NMPC_Delta_DOI_H2_Weight  IndexOptions=Index vector (dialog)  Indices=1  OutputSizes=1
  Data Store Read8 : DataStoreRead  DataStoreName=C2C_NMPC_DOI_Main_Weight  IndexOptions=Index vector (dialog)  Indices=1  OutputSizes=1
  Data Store Read9 : DataStoreRead  DataStoreName=C2C_NMPC_P2M_Weight  IndexOptions=Index vector (dialog)  Indices=1  OutputSizes=1
  Delay{,1..3} (4 alike) : Delay  DelayLength=1
  Demux{1..5} (5 alike) : Demux
  Discrete Derivative{1..4} (4 alike) : simulink/Discrete/Discrete Derivative  gainval=1.0  ICPrevScaledInput=0.0  OutMin=[]  OutMax=[]  OutDataType=fixdt(1, 16)  OutScaling=2^-10  DoSatur=off
  Discrete-Time Integrator : DiscreteIntegrator  SampleTime=-1  ICPrevOutput=DiscIntNeverNeededParam  ICPrevScaledInput=DiscIntNeverNeededParam
  Display{,1..16,18..21,23} (22 alike) : Display
  Gain : Gain  Gain=20
  Gain6 : Gain  Gain=5
  Product{,1..14,16..20} (20 alike) : Product
  Scope : Scope  NumInputPorts=4
  Scope1 : Scope  NumInputPorts=3
  Selector1 : Selector  IndexOptions=Index vector (dialog)  Indices=[5:8]  OutputSizes=1
  Selector2 : Selector  IndexOptions=Index vector (dialog)  Indices=[1:4]  OutputSizes=1
  Square1 : Math  Operator=square  SignedPower=on
  Square4 : Math  Operator=square  SignedPower=on
  Staging : Subsystem
  Subsystem : Subsystem
  Subsystem1 : Subsystem
  Subsystem2 : Subsystem
  Subsystem3 : Subsystem
  Subsystem4 : Subsystem
  Subsystem5 : Subsystem  Commented=on
  Subsystem6 : Subsystem  Commented=on
  Subtract{,1..3} (4 alike) : Sum  Inputs=+-
  Sum : Sum  Inputs=++++++
  Sum{1..5} (5 alike) : Sum  Inputs=++++
  TrackingError : Subsystem
  Cost : Outport  VectorParamsAs1DForOutWhenUnconnected=off
  wires:
  Sum/1 -> Cost/1
  Outputs/1 -> Display5/1, Demux1/1, TrackingError/1(Outputs), Display4/1, Staging/1(Output)
  Data Store Read/1 -> Product/1
  Data Store Read1/1 -> Product1/1
  Data Store Read2/1 -> Product2/1
  Data Store Read3/1 -> Product3/1
  Product2/1 -> Sum2/3
  Product1/1 -> Sum2/2
  Product/1 -> Sum2/1
  Product3/1 -> Sum2/4
  TrackingError/1(TrackingError) -> Square1/1, Display14/1
  Product4/1 -> Sum3/1
  Data Store Read10/1 -> Product6/1
  Product7/1 -> Sum3/4
  Product5/1 -> Sum3/2
  Data Store Read8/1 -> Product4/1
  ControlError/1(ControlError) -> Square4/1
  Data Store Read9/1 -> Product5/1
  Product6/1 -> Sum3/3
  Data Store Read11/1 -> Product7/1
  Sum2/1 -> Discrete-Time Integrator/1, Product8/1
  Data Store Read12/1 -> Product8/2
  Sum3/1 -> Product9/1
  Data Store Read13/1 -> Product9/2
  Square4/1 -> Demux3/1
  Data Store Read17/1 -> Product11/1
  Data Store Read15/1 -> Product13/1
  Demux4/2 -> Discrete Derivative2/1
  Demux4/1 -> Discrete Derivative1/1
  Product12/1 -> Abs7/1
  Product10/1 -> Display6/1, Abs5/1
  Product13/1 -> Abs8/1
  Demux4/4 -> Discrete Derivative4/1
  Demux4/3 -> Discrete Derivative3/1
  Data Store Read16/1 -> Product10/1
  Data Store Read14/1 -> Product12/1
  Product11/1 -> Abs6/1
  Discrete Derivative1/1 -> Product10/2
  Discrete Derivative2/1 -> Product11/2
  Discrete Derivative3/1 -> Product12/2
  Discrete Derivative4/1 -> Product13/2
  Data Store Read4/1 -> Product14/2
  Sum4/1 -> Product14/1
  Demux1/1 -> Display12/1, Subsystem1/3(Inputvalue)
  Sum5/1 -> Gain/1
  Product8/1 -> Scope1/1, Display2/1, Sum/2
  Product20/1 -> Display9/1, Display8/1
  Product9/1 -> Sum/3, Display3/1
  Refernce/1 -> Selector2/1, Selector1/1
  Selector2/1 -> Staging/2(Reference_Output), TrackingError/2(ReferenceOutputs)
  Subsystem/1(Out1) -> Subsystem1/1(UpperBound), Display10/1
  Subsystem/2(Out2) -> Display11/1, Subsystem1/2(Lowerbound)
  Subsystem/3(Out3) -> Subsystem2/1(UpperBound)
  Subsystem/4(Lowerbound) -> Subsystem2/2(Lowerbound)
  Subsystem/5(Out5) -> Subsystem3/1(UpperBound)
  Subsystem/6(Out6) -> Subsystem3/2(Lowerbound)
  Subsystem/7(Out7) -> Scope/1, Subsystem4/1(UpperBound)
  Subsystem/8(Out8) -> Scope/2, Subsystem4/2(Lowerbound)
  Product19/1 -> Sum1/4
  Product16/1 -> Display7/1, Sum1/1
  Abs/1 -> Product16/2
  Product18/1 -> Sum1/3
  Demux5/1 -> Subtract/1, Delay/1
  Product17/1 -> Sum1/2
  Data Store Read7/1 -> Product19/1
  Data Store Read6/1 -> Product18/1
  Abs3/1 -> Product19/2
  Data Store Read19/1 -> Product17/1
  Data Store Read18/1 -> Product16/1
  Sum1/1 -> Product20/1
  Data Store Read20/1 -> Product20/2
  Delay/1 -> Subtract/2
  Subtract/1 -> Abs/1
  Subtract1/1 -> Abs1/1
  Delay1/1 -> Subtract1/2
  Demux5/2 -> Subtract1/1, Delay1/1
  Abs1/1 -> Product17/2
  Demux5/3 -> Subtract2/1, Delay2/1
  Delay2/1 -> Subtract2/2
  Subtract2/1 -> Abs2/1
  Abs2/1 -> Product18/2
  Demux5/4 -> Subtract3/1, Delay3/1
  Delay3/1 -> Subtract3/2
  Subtract3/1 -> Abs3/1
  Product14/1 -> Display1/1
  controls/1 -> Display23/1, Demux4/1, Demux5/1, Display21/1, ControlError/2(Controls)
  Subsystem1/1(Outputvalue) -> Sum5/1
  Subsystem2/1(Outputvalue) -> Sum5/2
  Subsystem4/1(Outputvalue) -> Scope/3, Sum5/4
  Abs5/1 -> Sum4/1
  Abs6/1 -> Sum4/2
  Abs7/1 -> Sum4/3
  Abs8/1 -> Sum4/4
  Gain/1 -> Sum/1, Scope1/3, Display/1
  Discrete-Time Integrator/1 -> Gain6/1
  Gain6/1 -> Display13/1
  Square1/1 -> Display15/1, Demux2/1
  Demux1/2 -> Display18/1, Subsystem2/3(Inputvalue)
  Demux1/3 -> Subsystem3/3(Inputvalue), Display19/1
  Demux1/4 -> Scope/4, Subsystem4/3(Inputvalue), Display20/1
  Staging/1(Out1) -> Scope1/2, Display16/1, Sum/5
  Selector1/1 -> ControlError/1(ReferenceControls)
  Subsystem3/1(Outputvalue) -> Sum5/3
  Demux2/1 -> Product/2
  Demux2/2 -> Product1/2
  Demux2/3 -> Product2/2
  Demux2/4 -> Product3/2
  Demux3/1 -> Product4/2
  Demux3/2 -> Product5/2
  Demux3/3 -> Product6/2
  Demux3/4 -> Product7/2

== system H2DFRL_LExCI_env_PPO/Engine Model/offset_and_noise/CA50_generation/denormalizing_CA50 ==
  CA50_in : Inport
  Constant : Constant  Value=C2C_NMPC.Normalization.outputs.mean(4)
  Gain : Gain  Gain=C2C_NMPC.Normalization.outputs.std(4)
  Sum5 : Sum  Inputs=|++
  CA50 : Outport
  wires:
  CA50_in/1 -> Gain/1
  Gain/1 -> Sum5/1
  Constant/1 -> Sum5/2
  Sum5/1 -> CA50/1

== system H2DFRL_LExCI_env_PPO/Engine Model/offset_and_noise/CA50_generation/normalizing_CA50 ==
  CA50 : Inport
  Constant : Constant  Value=C2C_NMPC.Normalization.outputs.mean(4)
  Gain : Gain  Gain=1/C2C_NMPC.Normalization.outputs.std(4)
  Sum5 : Sum  Inputs=|+-
  CA50_out : Outport
  wires:
  CA50/1 -> Sum5/1
  Constant/1 -> Sum5/2
  Gain/1 -> CA50_out/1
  Sum5/1 -> Gain/1

== system H2DFRL_LExCI_env_PPO/Engine Model/offset_and_noise/IMEP_generation/denormalizing_IMEP ==
  IMEP_in : Inport
  Constant : Constant  Value=C2C_NMPC.Normalization.outputs.mean(1)
  Gain : Gain  Gain=C2C_NMPC.Normalization.outputs.std(1)
  Sum5 : Sum  Inputs=|++
  IMEP : Outport
  wires:
  IMEP_in/1 -> Gain/1
  Gain/1 -> Sum5/1
  Constant/1 -> Sum5/2
  Sum5/1 -> IMEP/1

== system H2DFRL_LExCI_env_PPO/Engine Model/offset_and_noise/IMEP_generation/normalizing_IMEP ==
  IMEP : Inport
  Constant : Constant  Value=C2C_NMPC.Normalization.outputs.mean(1)
  Gain : Gain  Gain=1/C2C_NMPC.Normalization.outputs.std(1)
  Sum5 : Sum  Inputs=|+-
  IMEP_out : Outport
  wires:
  IMEP/1 -> Sum5/1
  Constant/1 -> Sum5/2
  Gain/1 -> IMEP_out/1
  Sum5/1 -> Gain/1

== system H2DFRL_LExCI_env_PPO/Engine Model/offset_and_noise1/IMEP_generation/denormalizing_IMEP ==
  IMEP_in : Inport
  Constant : Constant  Value=C2C_NMPC.Normalization.outputs.mean(1)
  Gain : Gain  Gain=C2C_NMPC.Normalization.outputs.std(1)
  Sum5 : Sum  Inputs=|++
  IMEP : Outport
  wires:
  IMEP_in/1 -> Gain/1
  Gain/1 -> Sum5/1
  Constant/1 -> Sum5/2
  Sum5/1 -> IMEP/1

== system H2DFRL_LExCI_env_PPO/Engine Model/offset_and_noise1/IMEP_generation/normalizing_IMEP ==
  IMEP : Inport
  Constant : Constant  Value=C2C_NMPC.Normalization.outputs.mean(1)
  Gain : Gain  Gain=1/C2C_NMPC.Normalization.outputs.std(1)
  Sum5 : Sum  Inputs=|+-
  IMEP_out : Outport
  wires:
  IMEP/1 -> Sum5/1
  Constant/1 -> Sum5/2
  Gain/1 -> IMEP_out/1
  Sum5/1 -> Gain/1

== system H2DFRL_LExCI_env_PPO/RL_Block/RL_Agent/Sampling/Continuous Action ==
  norm_action_dist : Inport
  b_training_active : Inport  Port=2
  rl_algorithm_selector : Inport  Port=3
  ddpg_standard_deviation : Inport  Port=4
  Enable : EnablePort
  DDPG_Sampler : Subsystem
  Ground : Ground
  Multiport Switch : MultiPortSwitch  SaturateOnIntegerOverflow=off  InputSameDT=off
  PPO_Sampler : Subsystem
  "norm_action " : Outport
  wires:
  rl_algorithm_selector/1 -> Multiport Switch/1
  norm_action_dist/1 -> DDPG_Sampler/1(norm_action_dist), PPO_Sampler/1(norm_action_dist)
  b_training_active/1 -> PPO_Sampler/2(b_training_active), DDPG_Sampler/2(b_training_active)
  PPO_Sampler/1("norm_action ") -> Multiport Switch/2
  ddpg_standard_deviation/1 -> DDPG_Sampler/3(standard_deviation)
  DDPG_Sampler/1("norm_action ") -> Multiport Switch/3
  Ground/1 -> Multiport Switch/4
  Multiport Switch/1 -> "norm_action "/1

== system H2DFRL_LExCI_env_PPO/RL_Block/RL_Agent/Sampling/Discrete Action ==
  note: Distribute into single actions
  note: Softmax
  note: Allocate to discrete action
  note: Warning, if discrete action is selected alongside with DDPG.
  note: Not implemented yet.
  norm_action_dist : Inport
  b_training_active : Inport  Port=2
  rl_algorithm_selector : Inport  Port=3
  Enable : EnablePort
  Action Mean Selector : Constant  Commented=on  Value=1:1:NUMBER_OF_ACTIONS  OutDataTypeStr=single
  Ground : Ground
  Mean Selector : Selector  Commented=on  InputPortWidth=2*NUMBER_OF_ACTIONS  IndexOptions=Index vector (port)  Indices=1  OutputSizes=1
  Terminator : Terminator  Commented=on
  Terminator1 : Terminator
  Terminator2 : Terminator
  Terminator3 : Terminator
  "norm_action " : Outport
  wires:
  Action Mean Selector/1 -> Mean Selector/2
  norm_action_dist/1 -> Terminator1/1
  Mean Selector/1 -> Terminator/1
  Ground/1 -> "norm_action "/1
  b_training_active/1 -> Terminator2/1
  rl_algorithm_selector/1 -> Terminator3/1

== system H2DFRL_LExCI_env_PPO/Signal Processing/calculate reward/Subsystem/ControlError ==
  ReferenceControls : Inport
  Controls : Inport  Port=2
  Demux1 : Demux
  Demux2 : Demux
  Mux : Mux
  Subtract{,1..3} (4 alike) : Sum  Inputs=+-
  ControlError : Outport
  wires:
  Demux2/4 -> Subtract3/2
  Demux1/2 -> Subtract1/1
  Demux1/1 -> Subtract/1
  Demux2/2 -> Subtract1/2
  Demux2/3 -> Subtract2/2
  Controls/1 -> Demux2/1
  Demux1/3 -> Subtract2/1
  Demux1/4 -> Subtract3/1
  Demux2/1 -> Subtract/2
  Mux/1 -> ControlError/1
  Subtract/1 -> Mux/1
  Subtract1/1 -> Mux/2
  Subtract2/1 -> Mux/3
  Subtract3/1 -> Mux/4
  ReferenceControls/1 -> Demux1/1

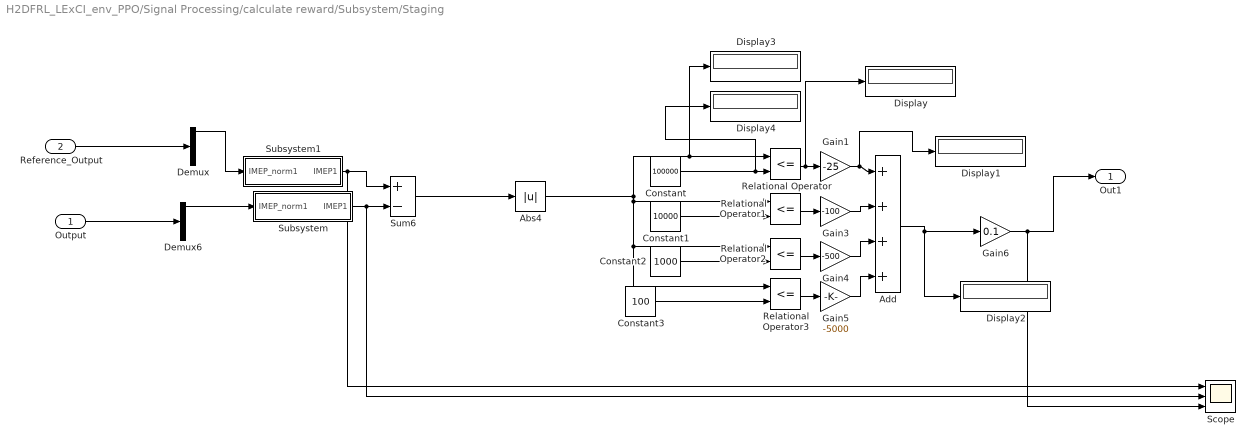
== system H2DFRL_LExCI_env_PPO/Signal Processing/calculate reward/Subsystem/Staging ==
  Output : Inport
  Reference_Output : Inport  Port=2
  Abs4 : Abs  SaturateOnIntegerOverflow=off
  Add : Sum  Inputs=++++
  Constant : Constant  Value=100000
  Constant1 : Constant  Value=10000
  Constant2 : Constant  Value=1000
  Constant3 : Constant  Value=100
  Demux : Demux
  Demux6 : Demux
  Display{,1..4} (5 alike) : Display
  Gain1 : Gain  Gain=-25
  Gain3 : Gain  Gain=-100
  Gain4 : Gain  Gain=-500
  Gain5 : Gain  Gain=-5000
  Gain6 : Gain  Gain=0.1
  Relational Operator{,1..3} (4 alike) : RelationalOperator  Operator=<=  OutDataTypeStr=boolean  RndMeth=Simplest  InputSameDT=off
  Scope : Scope  NumInputPorts=3
  Subsystem : Subsystem
  Subsystem1 : Subsystem
  Sum6 : Sum  Inputs=+-
  Out1 : Outport
  wires:
  Reference_Output/1 -> Demux/1
  Gain5/1 -> Add/4
  Gain4/1 -> Add/3
  Relational Operator1/1 -> Gain3/1
  Demux6/1 -> Subsystem/1(IMEP_norm1)
  Gain3/1 -> Add/2
  Relational Operator3/1 -> Gain5/1
  Demux/1 -> Subsystem1/1(IMEP_norm1)
  Output/1 -> Demux6/1
  Relational Operator2/1 -> Gain4/1
  Add/1 -> Display2/1, Gain6/1
  Relational Operator/1 -> Display/1, Gain1/1
  Abs4/1 -> Display3/1, Relational Operator/1, Relational Operator1/1, Relational Operator2/1, Relational Operator3/1
  Sum6/1 -> Abs4/1
  Gain1/1 -> Display1/1, Add/1
  Constant3/1 -> Relational Operator3/2
  Constant2/1 -> Relational Operator2/2
  Constant1/1 -> Relational Operator1/2
  Constant/1 -> Display4/1, Relational Operator/2
  Gain6/1 -> Scope/3, Out1/1
  Subsystem/1(IMEP1) -> Scope/2, Sum6/2
  Subsystem1/1(IMEP1) -> Sum6/1, Scope/1
